simulink model "SideSlipController"  (Simulink 8.5)
settings: Solver=ode45  StartTime=0  StopTime=50.0  FixedStep=1  RelTol=1e-3
libraries: simulink x3
settings Model: Creator=Suriya  LastModifiedBy=spachaimuthu
settings DebuggingCC: SolverPrmCheckMsg=warning  FcnCallInpInsideContextMsg=EnableAllAsWarning
settings GRTTargetCC: CombineOutputUpdateFcns=on  GRTInterface=off

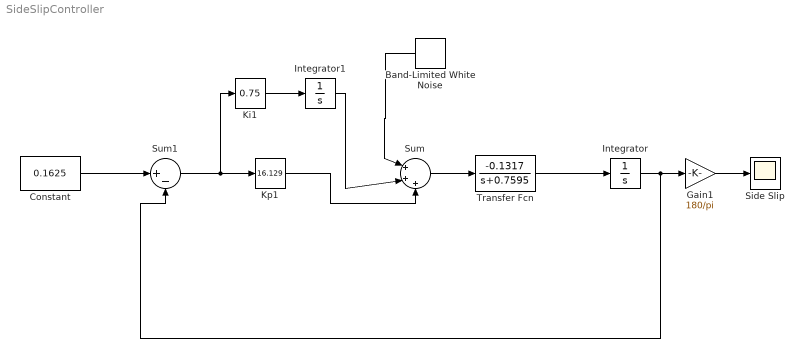
== system SideSlipController ==
  Band-Limited White Noise : simulink/Sources/Band-Limited White Noise  Cov=[0.1]  Ts=0.1  seed=[23341]
  Constant : Constant  Value=0.1625
  Gain1 : Gain  Gain=180/pi
  Integrator : Integrator
  Integrator1 : Integrator
  Ki1 : simulink/Math Operations/Slider Gain  low=0  gain=0.75  high=200
  Kp1 : simulink/Math Operations/Slider Gain  low=0  gain=16.129  high=500
  Side Slip : Scope
  Sum : Sum  Inputs=|+++
  Sum1 : Sum  Inputs=|+-
  Transfer Fcn : TransferFcn  Numerator=[-0.1317]  Denominator=[1 0.7595]
  wires:
  Sum/1 -> Transfer Fcn/1
  Ki1/1 -> Integrator1/1
  Transfer Fcn/1 -> Integrator/1
  Band-Limited White Noise/1 -> Sum/1
  Integrator1/1 -> Sum/2
  Kp1/1 -> Sum/3
  Sum1/1 -> Kp1/1, Ki1/1
  Integrator/1 -> Gain1/1, Sum1/2
  Constant/1 -> Sum1/1
  Gain1/1 -> Side Slip/1
